simulink model "RW_model"  (R2023a)
settings: Solver=VariableStepAuto  StartTime=0.0  StopTime=100  RelTol=1e-3
undefined symbols (not defined in the file): B, J, Ke, Kt, La, Ra, T_max
settings Model: Creator=Personal  LastModifiedBy=Personal

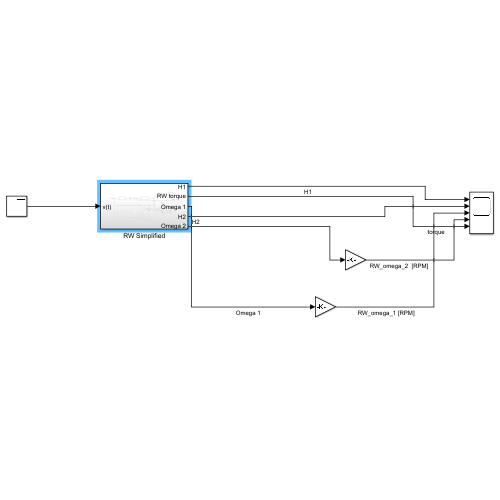
[thumbnail: Simulink's stored preview of the top-level diagram]
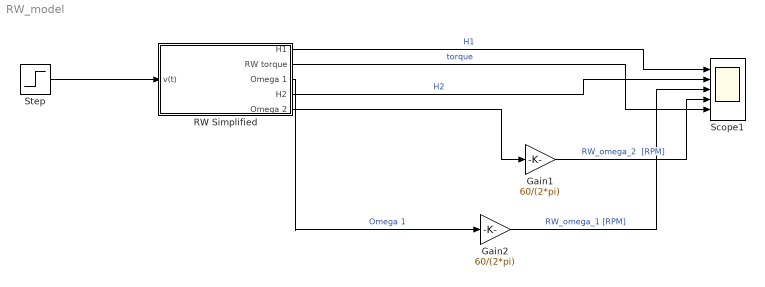
== system RW_model ==
  Gain1 : Gain  Gain=60/(2*pi)
  Gain2 : Gain  Gain=60/(2*pi)
  RW Simplified : Subsystem
  Scope1 : Scope  NumInputPorts=5
  Step : Step  Time=5  After=1e-3  SampleTime=0
  wires:
  RW Simplified/1(H1) -> Scope1/1  "H1"
  RW Simplified/2(RW torque) -> Scope1/5  "torque"
  RW Simplified/4(H2) -> Scope1/2  "H2"
  Step/1 -> RW Simplified/1(v(t))
  RW Simplified/5(Omega 2) -> Gain1/1
  Gain1/1 -> Scope1/4  "RW_omega_2  [RPM]"
  RW Simplified/3(Omega 1) -> Gain2/1  "Omega 1"
  Gain2/1 -> Scope1/3  "RW_omega_1 [RPM]"

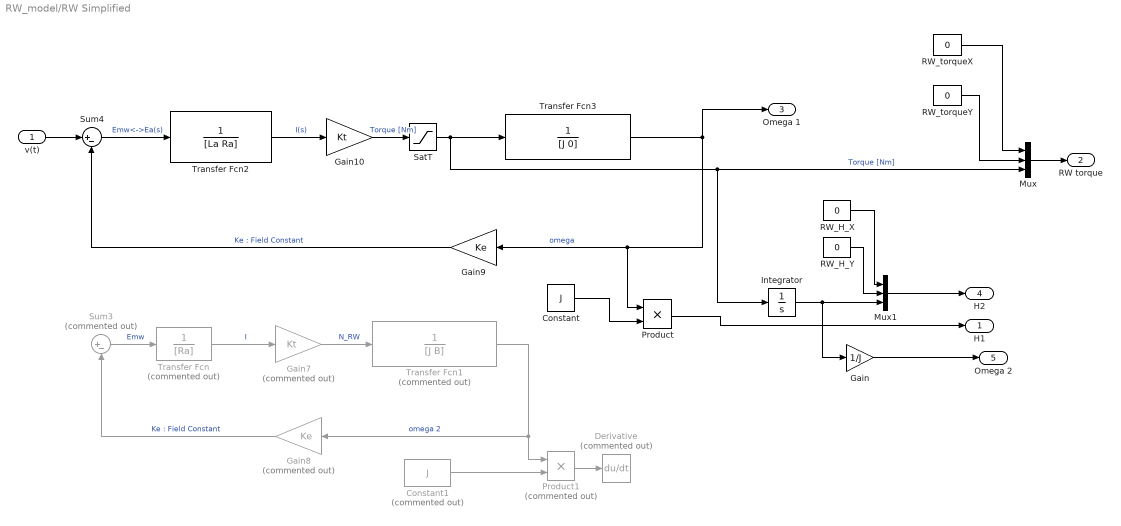
== system RW_model/RW Simplified ==
  v(t) : Inport
  Constant : Constant  Value=J
  Constant1 : Constant  Commented=on  Value=J
  Derivative : Derivative  Commented=on
  Gain : Gain  Gain=1/J
  Gain10 : Gain  Gain=Kt
  Gain7 : Gain  Commented=on  Gain=Kt
  Gain8 : Gain  Commented=on  Gain=Ke
  Gain9 : Gain  Gain=Ke
  Integrator : Integrator
  Mux : Mux  Inputs=3
  Mux1 : Mux  Inputs=3
  Product : Product
  Product1 : Product  Commented=on
  RW_H_X : Constant  Value=0
  RW_H_Y : Constant  Value=0
  RW_torqueX : Constant  Value=0
  RW_torqueY : Constant  Value=0
  SatT : Saturate  UpperLimit=T_max  LowerLimit=-T_max
  Sum3 : Sum  Commented=on  Inputs=|+-
  Sum4 : Sum  Inputs=|+-
  Transfer Fcn : TransferFcn  Commented=on  Denominator=[Ra]
  Transfer Fcn1 : TransferFcn  Commented=on  Denominator=[J B]
  Transfer Fcn2 : TransferFcn  Denominator=[La Ra]
  Transfer Fcn3 : TransferFcn  Denominator=[J 0]
  H1 : Outport  VectorParamsAs1DForOutWhenUnconnected=off
  RW torque : Outport  Port=2  VectorParamsAs1DForOutWhenUnconnected=off
  Omega 1 : Outport  Port=3  VectorParamsAs1DForOutWhenUnconnected=off
  H2 : Outport  Port=4  VectorParamsAs1DForOutWhenUnconnected=off
  Omega 2 : Outport  Port=5  VectorParamsAs1DForOutWhenUnconnected=off
  wires:
  Transfer Fcn2/1 -> Gain10/1  "I(s)"
  Sum4/1 -> Transfer Fcn2/1  "Emw<->Ea(s)"
  Gain9/1 -> Sum4/2  "Ke : Field Constant"
  Transfer Fcn3/1 -> Gain9/1, Product/1, Omega 1/1  "omega"
  Constant/1 -> Product/2
  Integrator/1 -> Gain/1, Mux1/3
  v(t)/1 -> Sum4/1
  Product1/1 -> Derivative/1
  Constant1/1 -> Product1/2
  Transfer Fcn1/1 -> Product1/1, Gain8/1  "omega 2"
  Gain7/1 -> Transfer Fcn1/1  "N_RW"
  Sum3/1 -> Transfer Fcn/1  "Emw"
  Transfer Fcn/1 -> Gain7/1  "I"
  Gain8/1 -> Sum3/2  "Ke : Field Constant"
  RW_H_X/1 -> Mux1/1
  RW_H_Y/1 -> Mux1/2
  Mux1/1 -> H2/1
  RW_torqueX/1 -> Mux/1
  RW_torqueY/1 -> Mux/2
  Mux/1 -> RW torque/1
  Gain10/1 -> SatT/1  "Torque [Nm]"
  SatT/1 -> Integrator/1, Mux/3, Transfer Fcn3/1  "Torque [Nm]"
  Product/1 -> H1/1
  Gain/1 -> Omega 2/1
